simulink model "MBD_Prob2"  (R2020a)
settings: Solver=VariableStepAuto  StartTime=0.0  StopTime=100.0  RelTol=1e-3
model workspace (MAT data in the model file):
  K1 = 80000
  K2 = 500000
  M1 = 2500
  M2 = 320
  b = 350
settings Model: Creator=Noel Varghese  LastModifiedBy=Noel Varghese

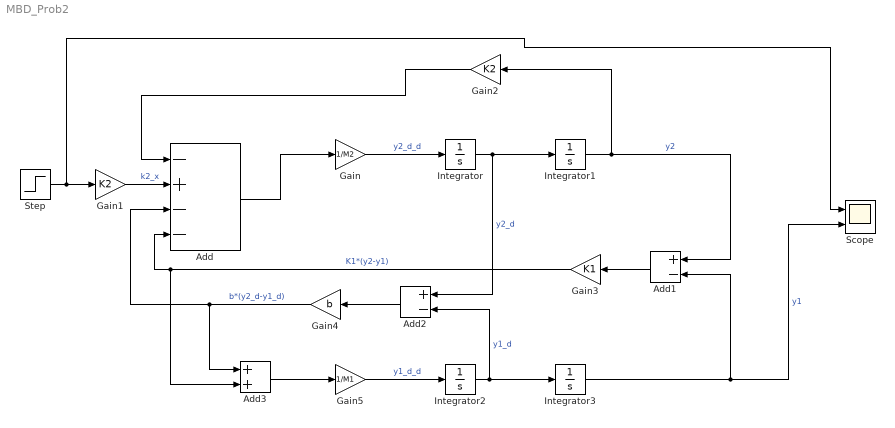
== system MBD_Prob2 ==
  Add : Sum  Inputs=-+--
  Add1 : Sum  Inputs=+-
  Add2 : Sum  Inputs=+-
  Add3 : Sum
  Gain : Gain  Gain=1/M2
  Gain1 : Gain  Gain=K2
  Gain2 : Gain  Gain=K2
  Gain3 : Gain  Gain=K1
  Gain4 : Gain  Gain=b
  Gain5 : Gain  Gain=1/M1
  Integrator{,1..3} (4 alike) : Integrator
  Scope : Scope  NumInputPorts=2
  Step : Step  SampleTime=0
  wires:
  Integrator/1 -> Add2/1, Integrator1/1  "y2_d"
  Gain/1 -> Integrator/1  "y2_d_d"
  Integrator1/1 -> Add1/1, Gain2/1  "y2"
  Add/1 -> Gain/1
  Step/1 -> Scope/1, Gain1/1
  Gain1/1 -> Add/2  "k2_x"
  Gain2/1 -> Add/1
  Integrator2/1 -> Add2/2, Integrator3/1  "y1_d"
  Gain5/1 -> Integrator2/1  "y1_d_d"
  Integrator3/1 -> Scope/2, Add1/2  "y1"
  Gain3/1 -> Add3/2, Add/4  "K1*(y2-y1)"
  Add1/1 -> Gain3/1
  Add2/1 -> Gain4/1
  Gain4/1 -> Add3/1, Add/3  "b*(y2_d-y1_d)"
  Add3/1 -> Gain5/1
